simulink model "battery_model"  (R2023a)
settings: Solver=VariableStepAuto  StartTime=0.0  StopTime=10.0  RelTol=1e-3
settings Model: Creator=Pedro  LastModifiedBy=Pedro

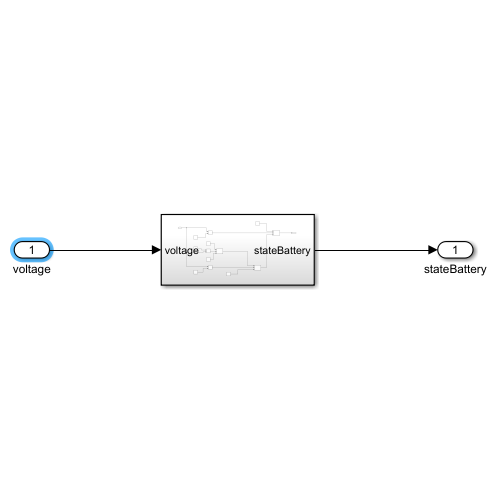
[thumbnail: Simulink's stored preview of the top-level diagram]
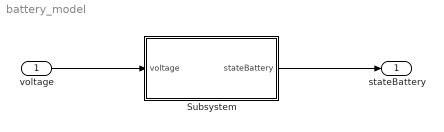
== system battery_model ==
  voltage : Inport
  Subsystem : Subsystem
  stateBattery : Outport
  wires:
  voltage/1 -> Subsystem/1(voltage)
  Subsystem/1(stateBattery) -> stateBattery/1

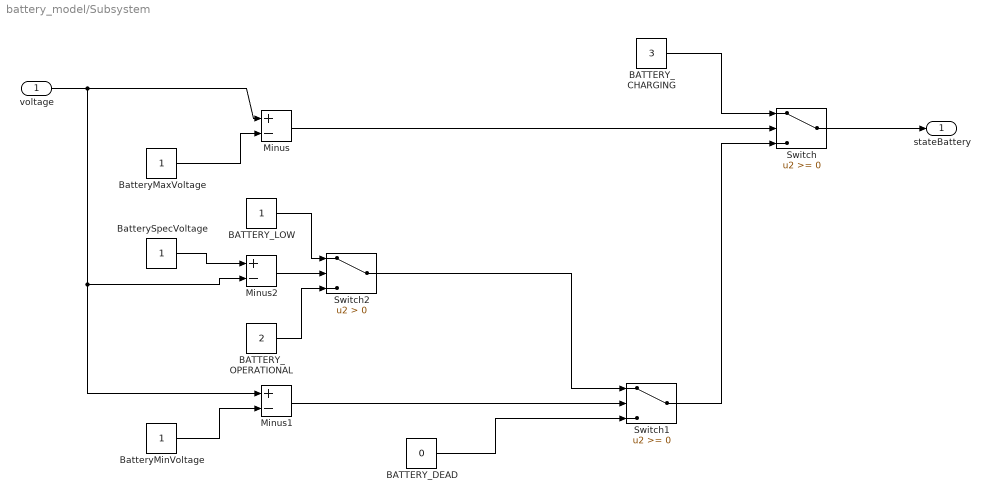
== system battery_model/Subsystem ==
  voltage : Inport
  BATTERY_CHARGING : Constant  Value=3
  BATTERY_DEAD : Constant  Value=0
  BATTERY_LOW : Constant
  BATTERY_OPERATIONAL : Constant  Value=2
  BatteryMaxVoltage : Constant
  BatteryMinVoltage : Constant
  BatterySpecVoltage : Constant
  Minus : Sum  Inputs=+-
  Minus1 : Sum  Inputs=+-
  Minus2 : Sum  Inputs=+-
  Switch : Switch  SaturateOnIntegerOverflow=off  InputSameDT=off
  Switch1 : Switch  SaturateOnIntegerOverflow=off  InputSameDT=off
  Switch2 : Switch  Criteria=u2 > Threshold  SaturateOnIntegerOverflow=off  InputSameDT=off
  stateBattery : Outport
  wires:
  Switch2/1 -> Switch1/1
  BATTERY_OPERATIONAL/1 -> Switch2/3
  BATTERY_CHARGING/1 -> Switch/1
  Minus2/1 -> Switch2/2
  Minus/1 -> Switch/2
  BatteryMaxVoltage/1 -> Minus/2
  voltage/1 -> Minus2/2, Minus1/1, Minus/1
  BatteryMinVoltage/1 -> Minus1/2
  BATTERY_DEAD/1 -> Switch1/3
  Switch1/1 -> Switch/3
  BATTERY_LOW/1 -> Switch2/1
  Minus1/1 -> Switch1/2
  Switch/1 -> stateBattery/1
  BatterySpecVoltage/1 -> Minus2/1
